simulink model "PID_earth"  (Simulink 6.0)
settings: Solver=ode23  StartTime=0.0  StopTime=100  RelTol=1e-8
undefined symbols (not defined in the file): B, DL, DQ, I, m, M, rg, slcm, T, W, xb, xg, Xudot, yb, yg, Yvdot, zb, zg, Zwdot
libraries: simulink_extras x4, rov_design_analysis x1
settings Model: LastModifiedBy=c chin

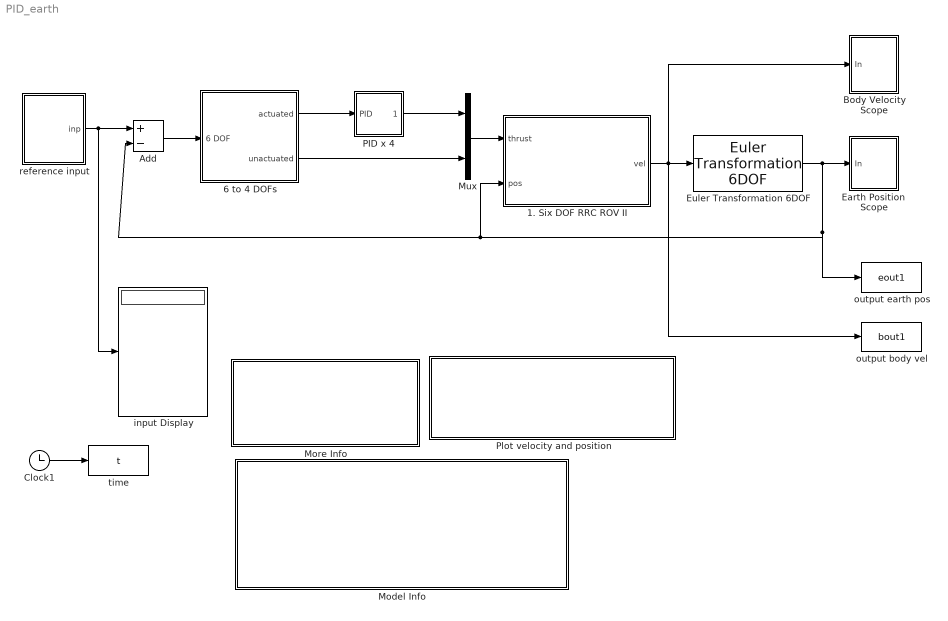
== system PID_earth ==
  " PID x 4" : Subsystem  AncestorBlock=|
      | rov_design_analysis/ROV Controller
      | Design
      | Applications/8. PID x 4
  1. Six DOF RRC ROV II : Subsystem  AncestorBlock=rov_design_analysis/ROV Models/1. Six DOF RRC ROV II
      mask Display:
      | disp('ROV')
      | image(imread('/rov_design_analysis/fig/ROVRRC2.jpg'));
      | color('black');port_label('input',1,'thrust')
      | color('black');port_label('input',2,'pos')
      | color('black');port_label('output',1,'vel')
  6 to 4 DOFs : Subsystem  AncestorBlock=rov_design_analysis/Scope Utilities/6 to 4 DOFs
  Add : Sum  Inputs=+-  OutScaling=2^-10
  "Body Velocity Scope " : Subsystem  AncestorBlock=rov_design_analysis/Utilities/Body Velocity Scope
      mask Display: disp('Body\nVelocity\nScope')
  Clock1 : Clock
      settings: Decimation=10
  "Earth Position  Scope " : Subsystem  AncestorBlock="rov_design_analysis/Utilities/Earth Position  Scope"
      mask Display: disp('Earth\nPosition\nScope')
  Euler Transformation 6DOF : rov_design_analysis/Utilities/Euler Transformation 6DOF
  Model Info : Subsystem  LoadFcn=slcm LoadBlock;  InitFcn=slcm('UpdateAllCMBlocksInThisModelInit')  mask(CMBlock){InitialSaveTempField=, InitialBlockCM=None, BlockCM=None, Frame=on, SaveTempField=, DisplayStringWithTags=|, MaskDisplayString=Reference:\n\nRobust controller design method and stability\nanalysis of an underactuated underwater vehicle, \n\nInternational Journal of Applied Mathematics and \n Computer Science, Vol 16, No. 3, p101-112, Dec 2006.\n\nAuthor: C.S. Chin et. al.\n21-Feb-2008 09:06:10, HorizontalTextAlignment=Left, LeftAlignmentValue=0.02, SourceBlockDiagram=PID_earth, TagMaxNumber=20, CMTag1=, CMTag2=, CMTag3=, CMTag4=, CMTag5=, CMTag6=, CMTag7=, CMTag8=, CMTag9=, CMTag10=, CMTag11=, CMTag12=, CMTag13=, CMTag14=, CMTag15=, CMTag16=, CMTag17=, CMTag18=, CMTag19=, CMTag20=}
      mask DisplayStringWithTags=|
      | Reference:\n
      | Robust controller design method and stability
      | analysis of an underactuated underwater vehicle, \n
      | International Journal of Applied Mathematics and \n Computer Science, Vol 16, No. 3, p101-112, Dec 2006.\n
      | %<Creator>Author: C.S. Chin et. al.
      | %<LastModificationDate>
      mask help: This block allows revision control information to be displayed within the model.
      settings: CopyFcn=slcm CopyBlock;  DeleteFcn=slcm Cancel;  PostSaveFcn=slcm('UpdateAllCMBlocksInThisModel')  NameChangeFcn=slcm Rename;  OpenFcn=slcm
      mask Display: text(str2num(LeftAlignmentValue), 0.5, MaskDisplayString, 'HorizontalAlignment', HorizontalTextAlignment)
  More Info : Subsystem
      settings: OpenFcn=|
      | cd c:\Matlab7\toolbox\rov_design_analysis\\mat_file ;
      | load rrcrovf;
      | kp1=11;ki1=2;kd1=1; kp2=11;ki2=4;kd2=1;kp3=9;ki3=1;kd3=2;kp4=1;ki4=2;kd4=1;
      mask Display: disp('Double-click here \n to \n load parameters')
  Mux : Mux  Inputs=2
  Plot velocity and position : Subsystem
      settings: OpenFcn=|
      | clc
      | cd c:\Matlab7\toolbox\rov_design_analysis\\m_file ;
      | run nonlin_resp6
      mask Display: disp('Double-click \n to \n Plot Velocity \n and \n Position')
  input Display : Display
  output body vel : ToWorkspace  VariableName=bout1  SampleTime=1  SaveFormat=Array
  output earth pos : ToWorkspace  VariableName=eout1  SampleTime=1  SaveFormat=Array
  reference input : Subsystem  AncestorBlock=|
      | rov_design_analysis/Scope
      | Utilities/pipe tracking
      | profile 
      | (Manual)
  time : ToWorkspace  VariableName=t  SampleTime=1  SaveFormat=Array
  wires:
  Euler Transformation 6DOF/1 -> Add/2, 1. Six DOF RRC ROV II/2("pos "), output earth pos/1, "Earth Position  Scope "/1(In)
  Clock1/1 -> time/1
  Add/1 -> 6 to 4 DOFs/1(6 DOF)
  6 to 4 DOFs/1(actuated) -> " PID x 4"/1(PID)
  " PID x 4"/1(" ") -> Mux/1
  Mux/1 -> 1. Six DOF RRC ROV II/1("thrust ")
  6 to 4 DOFs/2(unactuated) -> Mux/2
  reference input/1(inp) -> Add/1, input Display/1
  1. Six DOF RRC ROV II/1(vel) -> output body vel/1, Euler Transformation 6DOF/1, "Body Velocity Scope "/1(In)

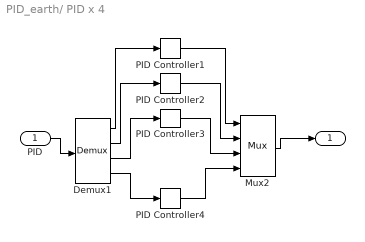
== system PID_earth/ PID x 4 ==
  PID : Inport  Port=1  LatchInput=off
  Demux1 : Demux
  Mux2 : Mux
  PID Controller1 : simulink_extras/Additional Linear/PID Controller  P=11  I=2  D=1
  PID Controller2 : simulink_extras/Additional Linear/PID Controller  P=11  I=4  D=1
  PID Controller3 : simulink_extras/Additional Linear/PID Controller  P=9  I=1  D=2
  PID Controller4 : simulink_extras/Additional Linear/PID Controller  P=1  I=2  D=1
  " " : Outport
  wires:
  Mux2/1 -> " "/1
  PID/1 -> Demux1/1
  PID Controller2/1 -> Mux2/2
  PID Controller1/1 -> Mux2/1
  Demux1/2 -> PID Controller2/1
  Demux1/1 -> PID Controller1/1
  Demux1/3 -> PID Controller3/1
  PID Controller3/1 -> Mux2/3
  Demux1/4 -> PID Controller4/1
  PID Controller4/1 -> Mux2/4

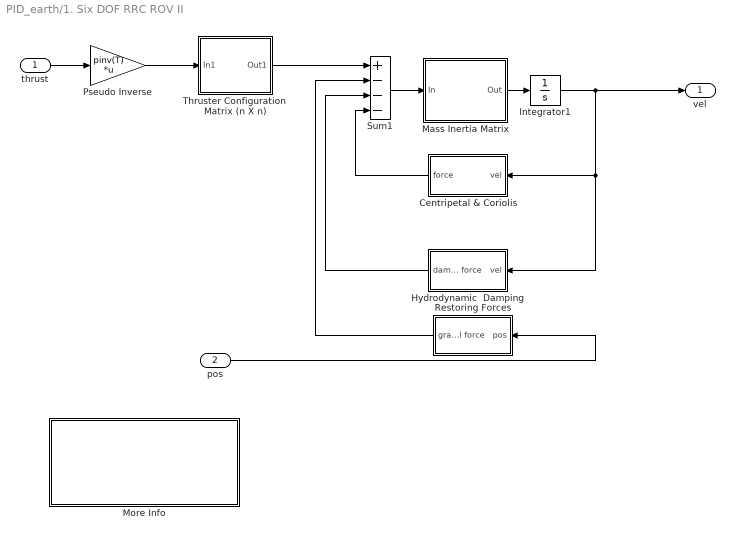
== system PID_earth/1. Six DOF RRC ROV II ==
  "thrust " : Inport  Port=1  LatchInput=off
  "pos " : Inport  Port=2  LatchInput=off
  Centripetal & Coriolis : Subsystem  Orientation=left
      mask Display: disp('Coriolis \n& Centrpetal \nMatrix')
  Hydrodynamic  Damping : Subsystem  Orientation=left
      mask Display: disp('Hydrodynamic \nDamping')
  Integrator1 : Integrator
  Mass Inertia Matrix : Subsystem
      mask Display: disp('Inverse Mass \n Inertia \n Matrix')
  More Info : Subsystem
      settings: OpenFcn=|
      | cd c:\Matlab7\toolbox\rov_design_analysis\\mat_file ;
      | load ROVRRC2;
      mask Display: disp('Double-click here to load the\n RRCROV2.mat')
  Pseudo Inverse : Gain  Gain=pinv(T)  Multiplication=Matrix(K*u)  SaturateOnIntegerOverflow=on
  Restoring Forces : Subsystem  Orientation=left
      mask Display: disp('Restoring\nForce')
  Sum1 : Sum  Inputs=+---  OutDataTypeMode=double  SaturateOnIntegerOverflow=on
  Thruster Configuration  Matrix (n X n) : Subsystem  AncestorBlock=|  mask(Thruster Configuration Matrix ){T=T}
      | rov_design_analysis/ROV
      | Models/4.  Thruster Configuration Matrix
      | (n X n)
      mask prompts: T "Insert Thruster Configuration Matrix"
      mask help: Provide the thruster configuration matrix using summation of forces and moment about the vehicle's C.G.
      mask Display: disp('Thruster \n Configuration')
  vel : Outport
  wires:
  Sum1/1 -> Mass Inertia Matrix/1(In)
  "pos "/1 -> Restoring Forces/1(pos)
  Centripetal & Coriolis/1(force) -> Sum1/4
  Hydrodynamic  Damping/1(damping force) -> Sum1/3
  Restoring Forces/1(gravitational force) -> Sum1/2
  Mass Inertia Matrix/1(Out) -> Integrator1/1
  Integrator1/1 -> vel/1, Centripetal & Coriolis/1(vel), Hydrodynamic  Damping/1(vel)
  Thruster Configuration  Matrix (n X n)/1(Out1) -> Sum1/1
  "thrust "/1 -> Pseudo Inverse/1
  Pseudo Inverse/1 -> Thruster Configuration  Matrix (n X n)/1(In1)

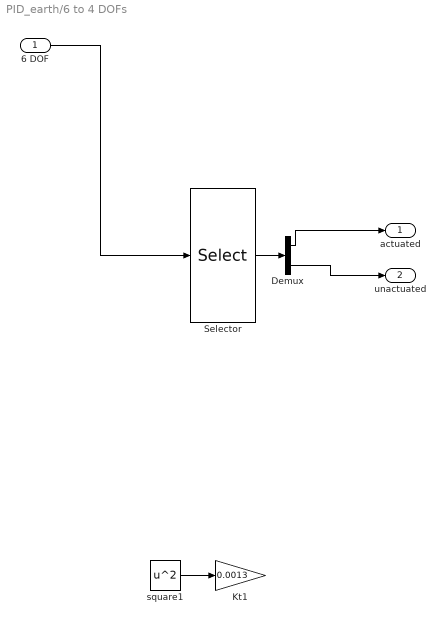
== system PID_earth/6 to 4 DOFs ==
  6 DOF : Inport  Port=1  LatchInput=off
  Demux : Demux  Outputs=2
  Kt1 : Gain  Gain=0.0013  SaturateOnIntegerOverflow=on
  Selector : Selector  Elements=[1 2 3 6 4 5]  InputPortWidth=6
  square1 : Math  Operator=square  SaturateOnIntegerOverflow=on
  actuated : Outport
  unactuated : Outport  Port=2
  wires:
  6 DOF/1 -> Selector/1
  square1/1 -> Kt1/1
  Selector/1 -> Demux/1
  Demux/1 -> actuated/1
  Demux/2 -> unactuated/1

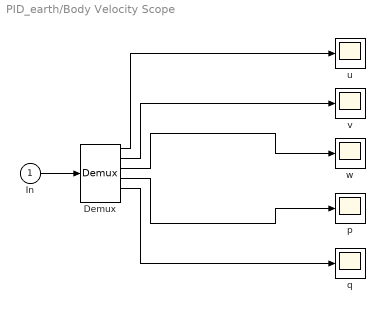
== system PID_earth/Body Velocity Scope  ==
  In : Inport  Port=1  LatchInput=off
  Demux : Demux  Outputs=6
  p : Scope
      settings: TickLabels=on  YMin=-0.125  YMax=0.2  DataFormat=Array
  q : Scope
      settings: TickLabels=on  TimeRange=200  YMin=-0.05  YMax=0.15  DataFormat=Array
  u : Scope
      settings: TickLabels=on  TimeRange=50  YMin=-0.025  YMax=0.375  DataFormat=Array
  v : Scope
      settings: TickLabels=on  YMin=-0.02  YMax=0.1  DataFormat=Array
  w : Scope
      settings: TickLabels=on  TimeRange=50  YMin=-0.0025  YMax=0.0375  DataFormat=Array
  wires:
  Demux/1 -> u/1
  Demux/2 -> v/1
  Demux/4 -> p/1
  Demux/3 -> w/1
  In/1 -> Demux/1
  Demux/5 -> q/1

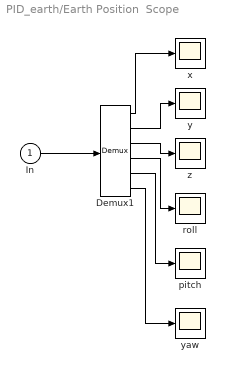
== system PID_earth/Earth Position  Scope  ==
  In : Inport  Port=1  LatchInput=off
  Demux1 : Demux  Outputs=6
  pitch : Scope
      settings: TickLabels=on  YMin=-0.05  YMax=0.15  DataFormat=Array
  roll : Scope
      settings: TickLabels=on  YMin=-0.125  YMax=0.2  DataFormat=Array
  x : Scope
      settings: TickLabels=on  TimeRange=50  YMin=0  YMax=0.375  DataFormat=Array
  y : Scope
      settings: TickLabels=on  YMin=-0.15  YMax=0.175  DataFormat=Array
  yaw : Scope
      settings: TickLabels=on  YMin=0  YMax=1.75  DataFormat=Array
  z : Scope
      settings: TickLabels=on  TimeRange=50  YMin=-0.0025  YMax=0.0375  DataFormat=Array
  wires:
  In/1 -> Demux1/1
  Demux1/1 -> x/1
  Demux1/6 -> yaw/1
  Demux1/5 -> pitch/1
  Demux1/4 -> roll/1
  Demux1/3 -> z/1
  Demux1/2 -> y/1

== system PID_earth/Model Info ==
  EmptySubsystem : Subsystem

== system PID_earth/More Info ==

== system PID_earth/Plot velocity and position ==

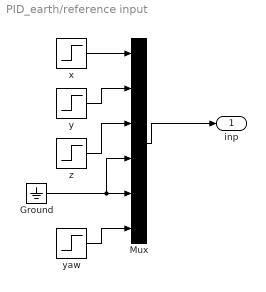
== system PID_earth/reference input ==
  Ground : Ground
  Mux : Mux  Inputs=6
  x : Step  Time=0  After=0.5  SampleTime=0
  y : Step  Time=0  After=0  SampleTime=0
  yaw : Step  Time=0  After=0  SampleTime=0
  z : Step  Time=0  SampleTime=0
  inp : Outport
  wires:
  x/1 -> Mux/1
  y/1 -> Mux/2
  z/1 -> Mux/3
  Mux/1 -> inp/1
  yaw/1 -> Mux/6
  Ground/1 -> Mux/4, Mux/5

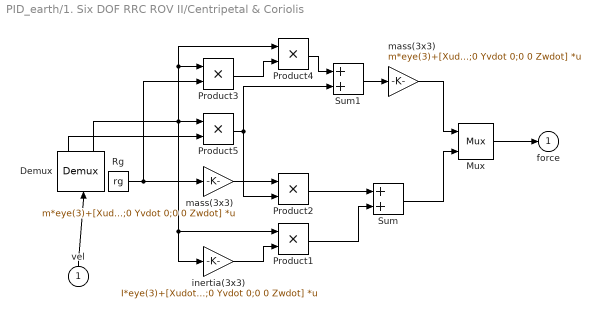
== system PID_earth/1. Six DOF RRC ROV II/Centripetal & Coriolis ==
  vel : Inport  Orientation=up  Port=1  LatchInput=off
  Demux : Demux  Orientation=up  Outputs=2
  Mux : Mux  Inputs=2
  Product{1..5} (5 alike) : Product  SaturateOnIntegerOverflow=on  RndMeth=Zero  InputSameDT=on
  Rg : Constant  Value=rg
  Sum : Sum  SaturateOnIntegerOverflow=on  InputSameDT=on
  Sum1 : Sum  SaturateOnIntegerOverflow=on  InputSameDT=on
  inertia(3x3) : Gain  Gain=I*eye(3)+[Xudot 0 0;0 Yvdot 0;0 0 Zwdot]  Multiplication=Matrix(K*u)  SaturateOnIntegerOverflow=on
  "mass(3x3) " : Gain  Gain=m*eye(3)+[Xudot 0 0;0 Yvdot 0;0 0 Zwdot]  Multiplication=Matrix(K*u)  SaturateOnIntegerOverflow=on
  "mass(3x3)   " : Gain  Gain=m*eye(3)+[Xudot 0 0;0 Yvdot 0;0 0 Zwdot]  Multiplication=Matrix(K*u)  SaturateOnIntegerOverflow=on
  force : Outport  InitialOutput=0
  wires:
  Product1/1 -> Sum/2
  "mass(3x3)   "/1 -> Product2/1
  Product2/1 -> Sum/1
  Rg/1 -> Product3/2, "mass(3x3)   "/1
  Product3/1 -> Product4/2
  Product4/1 -> Sum1/1
  Product5/1 -> Product2/2, Sum1/2
  Sum1/1 -> "mass(3x3) "/1
  Demux/2 -> Product5/1, Product3/1, Product4/1, Product1/1, inertia(3x3)/1
  Demux/1 -> Product5/2
  vel/1 -> Demux/1
  inertia(3x3)/1 -> Product1/2
  "mass(3x3) "/1 -> Mux/1
  Sum/1 -> Mux/2
  Mux/1 -> force/1

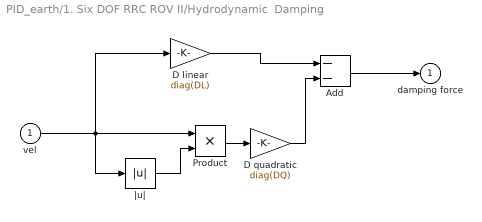
== system PID_earth/1. Six DOF RRC ROV II/Hydrodynamic  Damping ==
  vel : Inport  Port=1  LatchInput=off
  Add : Sum  Inputs=--  OutScaling=2^-10
  D linear : Gain  Gain=diag(DL)  SaturateOnIntegerOverflow=on
  D quadratic : Gain  Gain=diag(DQ)  SaturateOnIntegerOverflow=on
  Product : Product  SaturateOnIntegerOverflow=on  RndMeth=Zero  InputSameDT=on
  |u| : Abs  SaturateOnIntegerOverflow=on
  damping force : Outport  InitialOutput=0
  wires:
  Product/1 -> D quadratic/1
  D quadratic/1 -> Add/2
  vel/1 -> |u|/1, Product/1, D linear/1
  |u|/1 -> Product/2
  Add/1 -> damping force/1
  D linear/1 -> Add/1

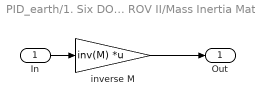
== system PID_earth/1. Six DOF RRC ROV II/Mass Inertia Matrix ==
  In : Inport  Port=1  LatchInput=off
  inverse M : Gain  Gain=inv(M)  Multiplication=Matrix(K*u)  SaturateOnIntegerOverflow=on
  Out : Outport
  wires:
  In/1 -> inverse M/1
  inverse M/1 -> Out/1

== system PID_earth/1. Six DOF RRC ROV II/More Info ==

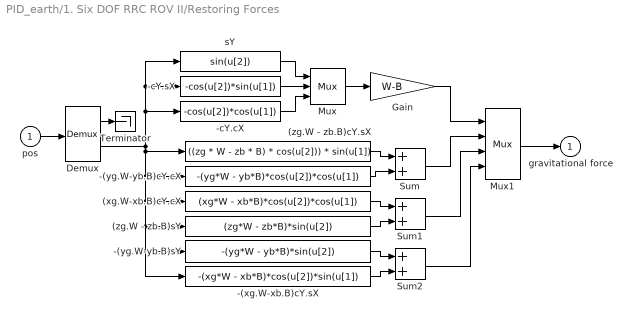
== system PID_earth/1. Six DOF RRC ROV II/Restoring Forces ==
  pos : Inport  Port=1  LatchInput=off
  (xg.W-xb.B)cY.cX : Fcn  Expr=(xg*W - xb*B)*cos(u[2])*cos(u[1])
  (zg.W - zb.B)cY.sX : Fcn  Expr=((zg * W - zb * B) * cos(u[2])) * sin(u[1])
  (zg.W - zb.B)sY : Fcn  Expr=(zg*W - zb*B)*sin(u[2])
  -(xg.W-xb.B)cY.sX : Fcn  Expr=-(xg*W - xb*B)*cos(u[2])*sin(u[1])
  -(yg.W-yb.B)cY.cX : Fcn  Expr=-(yg*W - yb*B)*cos(u[2])*cos(u[1])
  -(yg.W-yb.B)sY : Fcn  Expr=-(yg*W - yb*B)*sin(u[2])
  -cY.cX : Fcn  Expr=-cos(u[2])*cos(u[1])
  -cY.sX : Fcn  Expr=-cos(u[2])*sin(u[1])
  Demux : Demux  Outputs=2
  Gain : Gain  Gain=W-B  SaturateOnIntegerOverflow=on
  Mux : Mux  Inputs=3
  Mux1 : Mux
  Sum : Sum  SaturateOnIntegerOverflow=on  InputSameDT=on
  Sum1 : Sum  SaturateOnIntegerOverflow=on  InputSameDT=on
  Sum2 : Sum  SaturateOnIntegerOverflow=on  InputSameDT=on
  Terminator : Terminator
  sY : Fcn  Expr=sin(u[2])
  gravitational force : Outport  InitialOutput=0
  wires:
  pos/1 -> Demux/1
  Demux/1 -> Terminator/1
  Demux/2 -> -cY.cX/1, -cY.sX/1, sY/1, (zg.W - zb.B)cY.sX/1, -(yg.W-yb.B)cY.cX/1, (xg.W-xb.B)cY.cX/1, (zg.W - zb.B)sY/1, -(yg.W-yb.B)sY/1, -(xg.W-xb.B)cY.sX/1
  Mux1/1 -> gravitational force/1
  sY/1 -> Mux/1
  -cY.sX/1 -> Mux/2
  -cY.cX/1 -> Mux/3
  Mux/1 -> Gain/1
  Gain/1 -> Mux1/1
  -(yg.W-yb.B)cY.cX/1 -> Sum/2
  (zg.W - zb.B)cY.sX/1 -> Sum/1
  Sum/1 -> Mux1/2
  (zg.W - zb.B)sY/1 -> Sum1/2
  (xg.W-xb.B)cY.cX/1 -> Sum1/1
  Sum1/1 -> Mux1/3
  -(xg.W-xb.B)cY.sX/1 -> Sum2/2
  -(yg.W-yb.B)sY/1 -> Sum2/1
  Sum2/1 -> Mux1/4

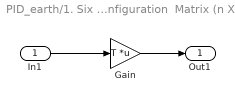
== system PID_earth/1. Six DOF RRC ROV II/Thruster Configuration  Matrix (n X n) ==
  In1 : Inport  Port=1  LatchInput=off
  Gain : Gain  Gain=T  Multiplication=Matrix(K*u)
  Out1 : Outport
  wires:
  In1/1 -> Gain/1
  Gain/1 -> Out1/1

== system PID_earth/Model Info/EmptySubsystem ==
